simulink model "RL_RC"  (R2016b)
settings: Solver=ode45  StartTime=0.05  StopTime=0.1  RelTol=1e-3  EnableMultiTasking=on
values from neighbouring files (symbols this model uses):
  K1 = 1/Leq    [untitledRLC.m]
  K2 = Req    [untitledRLC.m]
  K3 = 1/L1    (= 78.5398163397)    [untitledRLC.m]
  K4 = R1    (= 3)    [untitledRLC.m]
  K5 = 1/R2    (= 0.25)    [untitledRLC.m]
  K6 = C    (= 0.00106103295395)    [untitledRLC.m]
settings Model: Creator=الشاطئ  LastModifiedBy=HP
settings DataIOCC: LimitDataPoints=on  SaveFormat=Array
settings OptimizationCC: LifeSpan=inf
settings DebuggingCC: UnderspecifiedInitializationDetection=Classic  MergeDetectMultiDrivingBlocksExec=none  SolverPrmCheckMsg=warning  StateNameClashWarn=warning  SFUnexpectedBacktrackingDiag=warning  SFNoUnconditionalDefaultTransitionDiag=warning  SFExecutionAtInitializationDiag=none
settings HardwareCC: ProdBitPerPointer=32  ProdBitPerSizeT=32  ProdBitPerPtrDiffT=32  ProdLargestAtomicFloat=None  ProdIntDivRoundTo=Undefined  ProdEndianess=Unspecified  ProdWordSize=32  ProdHWDeviceType=32-bit Generic
settings ModelReferenceCC: PropagateSignalLabelsOutOfModel=off
settings GRTTargetCC: TargetLangStandard=C89/C90 (ANSI)  GeneratePreprocessorConditionals=Disable all
settings ConfigComp: CovMetricSettings=dw  CovHtmlReporting=on  CovSaveCumulativeToWorkspaceVar=on  CovSaveSingleToWorkspaceVar=on  CovExternalEMLEnable=off

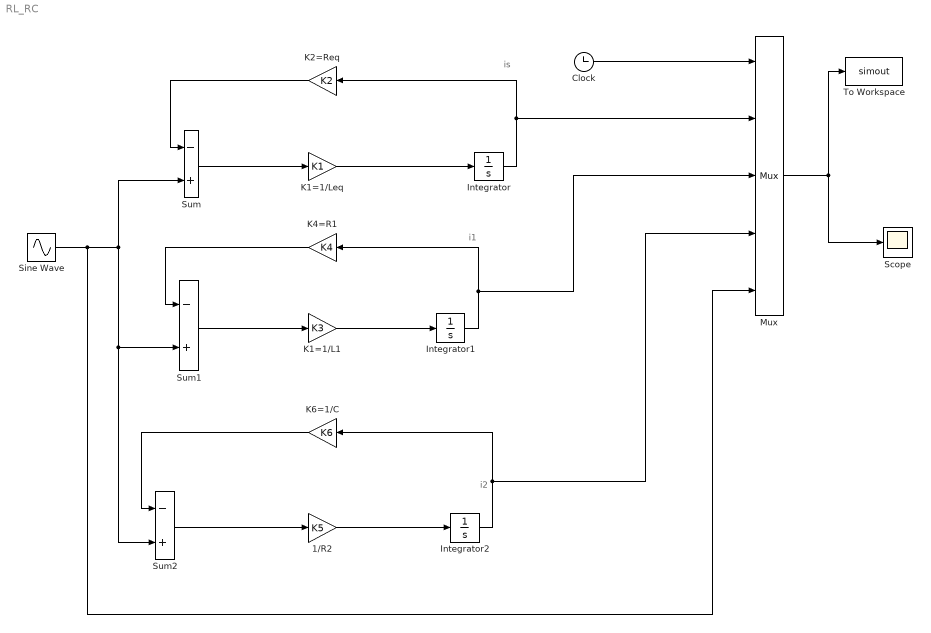
== system RL_RC ==
  note: i2
  note: i1
  note: is
  1/R2 : Gain  Gain=K5
  Clock : Clock
  Integrator : Integrator
  Integrator1 : Integrator
  Integrator2 : Integrator
  K1=1/L1 : Gain  Gain=K3
  K1=1/Leq : Gain  Gain=K1
  K2=Req : Gain  Gain=K2
  K4=R1 : Gain  Gain=K4
  K6=1/C : Gain  Gain=K6
  Mux : Mux  Inputs=5
  Scope : Scope
  Sine Wave : Sin  Amplitude=70  Frequency=2*pi*50  SampleTime=0
  Sum : Sum  Inputs=-+
  Sum1 : Sum  Inputs=-+
  Sum2 : Sum  Inputs=-+
  To Workspace : ToWorkspace  VariableName=simout  SampleTime=-1
  wires:
  Clock/1 -> Mux/1
  Sum/1 -> K1=1/Leq/1
  K1=1/Leq/1 -> Integrator/1
  Integrator/1 -> Mux/2, K2=Req/1
  K2=Req/1 -> Sum/1
  Sine Wave/1 -> Mux/5, Sum1/2, Sum2/2, Sum/2
  Sum1/1 -> K1=1/L1/1
  K1=1/L1/1 -> Integrator1/1
  Integrator1/1 -> K4=R1/1, Mux/3
  K4=R1/1 -> Sum1/1
  1/R2/1 -> Integrator2/1
  Integrator2/1 -> K6=1/C/1, Mux/4
  K6=1/C/1 -> Sum2/1
  Sum2/1 -> 1/R2/1
  Mux/1 -> Scope/1, To Workspace/1
